simulink model "Advanced_PID"  (R2023a)
settings: Solver=VariableStepAuto  StartTime=0.0  StopTime=100  RelTol=1e-3
model workspace (MAT data in the model file):
  A = [400000 0]
  Ti = 0
libraries: cstblocks x8, slpidlib x4
settings Model: PacingRate=5  Creator=munam  LastModifiedBy=Yuganshu Wadhwa

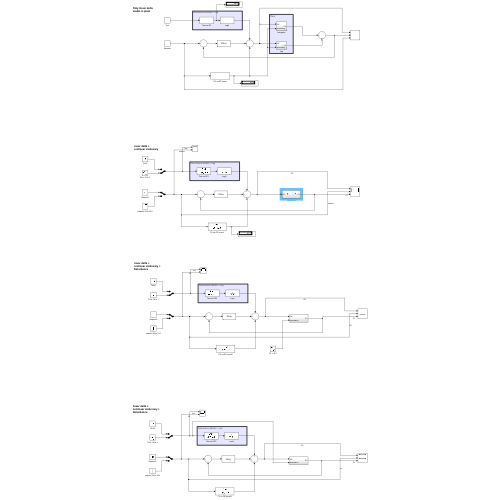
[thumbnail: Simulink's stored preview of the top-level diagram]
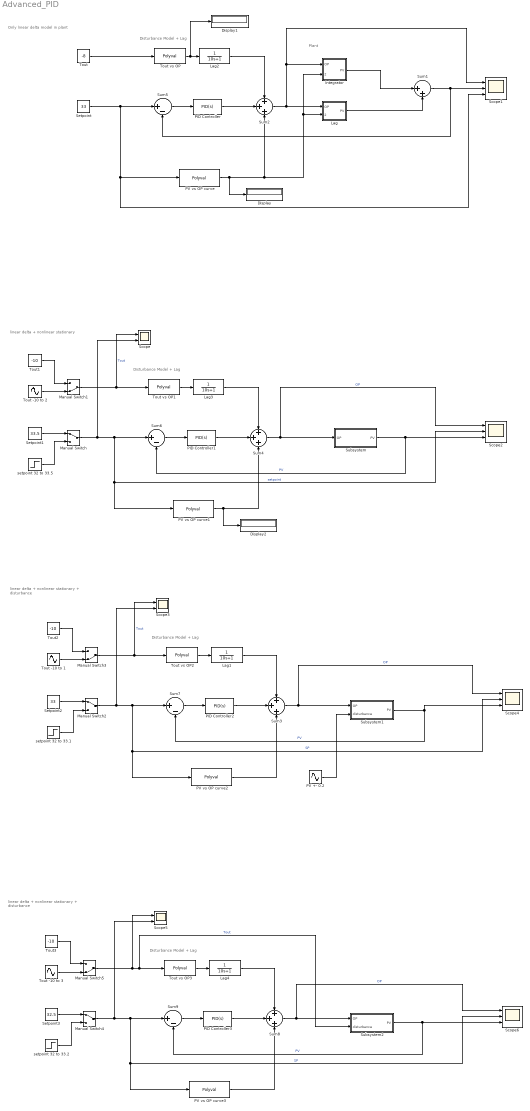
== system Advanced_PID ==
  note: Only linear delta model in plant
  note: Plant
  note: Disturbance Model + Lag
  note: Disturbance Model + Lag
  note: linear delta + nonlinear stationary
  note: linear delta + nonlinear stationary + disturbance
  note: Disturbance Model + Lag
  note: linear delta + nonlinear stationary + disturbance
  note: Disturbance Model + Lag
  Display : Display
  Display1 : Display
  Display2 : Display
  Integrator : Subsystem
  Lag : Subsystem
  Lag{1..4} (4 alike) : TransferFcn  Denominator=[10 1]
  Manual Switch : ManualSwitch
  Manual Switch1 : ManualSwitch  CurrentSetting=0
  Manual Switch2 : ManualSwitch
  Manual Switch3 : ManualSwitch  CurrentSetting=0
  Manual Switch4 : ManualSwitch
  Manual Switch5 : ManualSwitch  CurrentSetting=0
  PID Controller : slpidlib/PID Controller  Controller=PID  Form=Parallel  TimeDomain=Continuous-time  UseExternalTs=off  SampleTime=-1  IntegratorMethod=Forward Euler  FilterMethod=Forward Euler  ControllerParametersSource=internal  P=5  I=2  UseKiTs=off  D=0  N=1  UseFilter=on  TunerSelectOption=Transfer Function Based (PID Tuner App)  InitialConditionSource=internal  InitialConditionForIntegrator=0  InitialConditionForFilter=0  DifferentiatorICPrevScaledInput=0  ExternalReset=none  TrackingMode=off  Kt=1  LimitOutput=off  SatLimitsSource=internal  UpperSaturationLimit=100  LowerSaturationLimit=0  LinearizeAsGain=off  AntiWindupMode=none  Kb=1  LimitIntegrator=off  UpperIntegratorSaturationLimit=inf  LowerIntegratorSaturationLimit=-inf  POutMin=[]  POutMax=[]  IOutMin=[]  IOutMax=[]  DOutMin=[]  DOutMax=[]  NOutMin=[]  NOutMax=[]  SumOutMin=[]  SumOutMax=[]  SaturationOutMin=[]  SaturationOutMax=[]  PParamMin=[]  PParamMax=[]  IParamMin=[]  IParamMax=[]  DParamMin=[]  DParamMax=[]  NParamMin=[]  NParamMax=[]  KbParamMin=[]  KbParamMax=[]  KtParamMin=[]  KtParamMax=[]  KbOutMin=[]  KbOutMax=[]  KtOutMin=[]  KtOutMax=[]  IntegratorOutMin=[]  IntegratorOutMax=[]  FilterOutMin=[]  FilterOutMax=[]  SumI1OutMin=[]  SumI1OutMax=[]  SumI2OutMin=[]  SumI2OutMax=[]  SumI3OutMin=[]  SumI3OutMax=[]  SumI4OutMin=[]  SumI4OutMax=[]  SumDOutMin=[]  SumDOutMax=[]  DifferentiatorOutMin=[]  DifferentiatorOutMax=[]  FilterDiffOutCoefMin=[]  FilterDiffOutCoefMax=[]  ReciprocalOutMin=[]  ReciprocalOutMax=[]  SumDenOutMin=[]  SumDenOutMax=[]  SumNumOutMin=[]  SumNumOutMax=[]  DivideOutMin=[]  DivideOutMax=[]  UdiffTsProdOutMin=[]  UdiffTsProdOutMax=[]  NTsProdOutMin=[]  NTsProdOutMax=[]  UintegralTsProdOutMin=[]  UintegralTsProdOutMax=[]  UngainTsProdOutMin=[]  UngainTsProdOutMax=[]  ClampingZeroOutDataTypeStr=Inherit: Inherit via back propagation  ClampingZeroOutMin=[]  ClampingZeroOutMax=[]  FilterDenConstantOutDataTypeStr=Inherit: Inherit via back propagation  FilterDenConstantOutMin=[]  FilterDenConstantOutMax=[]  PCopyOutDataTypeStr=Inherit: Inherit via back propagation  PCopyOutMin=[]  PCopyOutMax=[]  NCopyOutDataTypeStr=Inherit: Inherit via back propagation  NCopyOutMin=[]  NCopyOutMax=[]  IntegratorContinuousStateAttributes=''  IntegratorStateMustResolveToSignalObject=off  IntegratorRTWStateStorageClass=Auto  FilterContinuousStateAttributes=''  FilterStateMustResolveToSignalObject=off  FilterRTWStateStorageClass=Auto  ParallelPVariant=InternalParameters  IdealPVariant=Disabled  IVariant=InternalParameters  DVariant=InternalParameters  IntegratorVariant=Continuous  SatVariant=Disabled  AWVariant=Passthrough  PCopyVariant=Disabled  TRVariant=Disabled  FdbkBlocksVariant=Forward  IdealPFdbkVariant=Disabled  SatFdbkVariant=Disabled  DerivativeFilterVariant=ContFilter  NVariant=InternalParameters  NCopyVariant=Disabled  FilterICVariant=InternalICsFilter  IntegratorICVariant=InternalICs  ExternalResetVariant=Disabled  TRSumVariant=Passthrough  SumFdbkVariant=Disabled  SumVariant=Sum_PID  TsampFilterVariant=InternalTs  TsampNgainVariant=Passthrough  TsampIntegralVariant=Disabled_SignalSpec  ExternalSaturationOutDataTypeStr=Inherit: Same as second input
  PID Controller1 : slpidlib/PID Controller  Controller=PID  Form=Parallel  TimeDomain=Continuous-time  UseExternalTs=off  SampleTime=-1  IntegratorMethod=Forward Euler  FilterMethod=Forward Euler  ControllerParametersSource=internal  P=5  I=3  UseKiTs=off  D=0  N=1  UseFilter=on  TunerSelectOption=Transfer Function Based (PID Tuner App)  InitialConditionSource=internal  InitialConditionForIntegrator=0  InitialConditionForFilter=0  DifferentiatorICPrevScaledInput=0  ExternalReset=none  TrackingMode=off  Kt=1  LimitOutput=off  SatLimitsSource=internal  UpperSaturationLimit=100  LowerSaturationLimit=0  LinearizeAsGain=off  AntiWindupMode=back-calculation  Kb=1  LimitIntegrator=off  UpperIntegratorSaturationLimit=inf  LowerIntegratorSaturationLimit=-inf  POutMin=[]  POutMax=[]  IOutMin=[]  IOutMax=[]  DOutMin=[]  DOutMax=[]  NOutMin=[]  NOutMax=[]  SumOutMin=[]  SumOutMax=[]  SaturationOutMin=[]  SaturationOutMax=[]  PParamMin=[]  PParamMax=[]  IParamMin=[]  IParamMax=[]  DParamMin=[]  DParamMax=[]  NParamMin=[]  NParamMax=[]  KbParamMin=[]  KbParamMax=[]  KtParamMin=[]  KtParamMax=[]  KbOutMin=[]  KbOutMax=[]  KtOutMin=[]  KtOutMax=[]  IntegratorOutMin=[]  IntegratorOutMax=[]  FilterOutMin=[]  FilterOutMax=[]  SumI1OutMin=[]  SumI1OutMax=[]  SumI2OutMin=[]  SumI2OutMax=[]  SumI3OutMin=[]  SumI3OutMax=[]  SumI4OutMin=[]  SumI4OutMax=[]  SumDOutMin=[]  SumDOutMax=[]  DifferentiatorOutMin=[]  DifferentiatorOutMax=[]  FilterDiffOutCoefMin=[]  FilterDiffOutCoefMax=[]  ReciprocalOutMin=[]  ReciprocalOutMax=[]  SumDenOutMin=[]  SumDenOutMax=[]  SumNumOutMin=[]  SumNumOutMax=[]  DivideOutMin=[]  DivideOutMax=[]  UdiffTsProdOutMin=[]  UdiffTsProdOutMax=[]  NTsProdOutMin=[]  NTsProdOutMax=[]  UintegralTsProdOutMin=[]  UintegralTsProdOutMax=[]  UngainTsProdOutMin=[]  UngainTsProdOutMax=[]  ClampingZeroOutDataTypeStr=Inherit: Inherit via back propagation  ClampingZeroOutMin=[]  ClampingZeroOutMax=[]  FilterDenConstantOutDataTypeStr=Inherit: Inherit via back propagation  FilterDenConstantOutMin=[]  FilterDenConstantOutMax=[]  PCopyOutDataTypeStr=Inherit: Inherit via back propagation  PCopyOutMin=[]  PCopyOutMax=[]  NCopyOutDataTypeStr=Inherit: Inherit via back propagation  NCopyOutMin=[]  NCopyOutMax=[]  IntegratorContinuousStateAttributes=''  IntegratorStateMustResolveToSignalObject=off  IntegratorRTWStateStorageClass=Auto  FilterContinuousStateAttributes=''  FilterStateMustResolveToSignalObject=off  FilterRTWStateStorageClass=Auto  ParallelPVariant=InternalParameters  IdealPVariant=Disabled  IVariant=InternalParameters  DVariant=InternalParameters  IntegratorVariant=Continuous  SatVariant=Disabled  AWVariant=Passthrough  PCopyVariant=Disabled  TRVariant=Disabled  FdbkBlocksVariant=Forward  IdealPFdbkVariant=Disabled  SatFdbkVariant=Disabled  DerivativeFilterVariant=ContFilter  NVariant=InternalParameters  NCopyVariant=Disabled  FilterICVariant=InternalICsFilter  IntegratorICVariant=InternalICs  ExternalResetVariant=Disabled  TRSumVariant=Passthrough  SumFdbkVariant=Disabled  SumVariant=Sum_PID  TsampFilterVariant=InternalTs  TsampNgainVariant=Passthrough  TsampIntegralVariant=Disabled_SignalSpec  ExternalSaturationOutDataTypeStr=Inherit: Same as second input
  PID Controller2 : slpidlib/PID Controller  Controller=PID  Form=Parallel  TimeDomain=Continuous-time  UseExternalTs=off  SampleTime=-1  IntegratorMethod=Forward Euler  FilterMethod=Forward Euler  ControllerParametersSource=internal  P=5  I=3  UseKiTs=off  D=0  N=1  UseFilter=on  TunerSelectOption=Transfer Function Based (PID Tuner App)  InitialConditionSource=internal  InitialConditionForIntegrator=0  InitialConditionForFilter=0  DifferentiatorICPrevScaledInput=0  ExternalReset=none  TrackingMode=off  Kt=1  LimitOutput=off  SatLimitsSource=internal  UpperSaturationLimit=100  LowerSaturationLimit=0  LinearizeAsGain=off  AntiWindupMode=back-calculation  Kb=1  LimitIntegrator=off  UpperIntegratorSaturationLimit=inf  LowerIntegratorSaturationLimit=-inf  POutMin=[]  POutMax=[]  IOutMin=[]  IOutMax=[]  DOutMin=[]  DOutMax=[]  NOutMin=[]  NOutMax=[]  SumOutMin=[]  SumOutMax=[]  SaturationOutMin=[]  SaturationOutMax=[]  PParamMin=[]  PParamMax=[]  IParamMin=[]  IParamMax=[]  DParamMin=[]  DParamMax=[]  NParamMin=[]  NParamMax=[]  KbParamMin=[]  KbParamMax=[]  KtParamMin=[]  KtParamMax=[]  KbOutMin=[]  KbOutMax=[]  KtOutMin=[]  KtOutMax=[]  IntegratorOutMin=[]  IntegratorOutMax=[]  FilterOutMin=[]  FilterOutMax=[]  SumI1OutMin=[]  SumI1OutMax=[]  SumI2OutMin=[]  SumI2OutMax=[]  SumI3OutMin=[]  SumI3OutMax=[]  SumI4OutMin=[]  SumI4OutMax=[]  SumDOutMin=[]  SumDOutMax=[]  DifferentiatorOutMin=[]  DifferentiatorOutMax=[]  FilterDiffOutCoefMin=[]  FilterDiffOutCoefMax=[]  ReciprocalOutMin=[]  ReciprocalOutMax=[]  SumDenOutMin=[]  SumDenOutMax=[]  SumNumOutMin=[]  SumNumOutMax=[]  DivideOutMin=[]  DivideOutMax=[]  UdiffTsProdOutMin=[]  UdiffTsProdOutMax=[]  NTsProdOutMin=[]  NTsProdOutMax=[]  UintegralTsProdOutMin=[]  UintegralTsProdOutMax=[]  UngainTsProdOutMin=[]  UngainTsProdOutMax=[]  ClampingZeroOutDataTypeStr=Inherit: Inherit via back propagation  ClampingZeroOutMin=[]  ClampingZeroOutMax=[]  FilterDenConstantOutDataTypeStr=Inherit: Inherit via back propagation  FilterDenConstantOutMin=[]  FilterDenConstantOutMax=[]  PCopyOutDataTypeStr=Inherit: Inherit via back propagation  PCopyOutMin=[]  PCopyOutMax=[]  NCopyOutDataTypeStr=Inherit: Inherit via back propagation  NCopyOutMin=[]  NCopyOutMax=[]  IntegratorContinuousStateAttributes=''  IntegratorStateMustResolveToSignalObject=off  IntegratorRTWStateStorageClass=Auto  FilterContinuousStateAttributes=''  FilterStateMustResolveToSignalObject=off  FilterRTWStateStorageClass=Auto  ParallelPVariant=InternalParameters  IdealPVariant=Disabled  IVariant=InternalParameters  DVariant=InternalParameters  IntegratorVariant=Continuous  SatVariant=Disabled  AWVariant=Passthrough  PCopyVariant=Disabled  TRVariant=Disabled  FdbkBlocksVariant=Forward  IdealPFdbkVariant=Disabled  SatFdbkVariant=Disabled  DerivativeFilterVariant=ContFilter  NVariant=InternalParameters  NCopyVariant=Disabled  FilterICVariant=InternalICsFilter  IntegratorICVariant=InternalICs  ExternalResetVariant=Disabled  TRSumVariant=Passthrough  SumFdbkVariant=Disabled  SumVariant=Sum_PID  TsampFilterVariant=InternalTs  TsampNgainVariant=Passthrough  TsampIntegralVariant=Disabled_SignalSpec  ExternalSaturationOutDataTypeStr=Inherit: Same as second input
  PID Controller3 : slpidlib/PID Controller  Controller=PID  Form=Parallel  TimeDomain=Continuous-time  UseExternalTs=off  SampleTime=-1  IntegratorMethod=Forward Euler  FilterMethod=Forward Euler  ControllerParametersSource=internal  P=5  I=3  UseKiTs=off  D=0  N=1  UseFilter=on  TunerSelectOption=Transfer Function Based (PID Tuner App)  InitialConditionSource=internal  InitialConditionForIntegrator=0  InitialConditionForFilter=0  DifferentiatorICPrevScaledInput=0  ExternalReset=none  TrackingMode=off  Kt=1  LimitOutput=off  SatLimitsSource=internal  UpperSaturationLimit=100  LowerSaturationLimit=0  LinearizeAsGain=off  AntiWindupMode=back-calculation  Kb=1  LimitIntegrator=off  UpperIntegratorSaturationLimit=inf  LowerIntegratorSaturationLimit=-inf  POutMin=[]  POutMax=[]  IOutMin=[]  IOutMax=[]  DOutMin=[]  DOutMax=[]  NOutMin=[]  NOutMax=[]  SumOutMin=[]  SumOutMax=[]  SaturationOutMin=[]  SaturationOutMax=[]  PParamMin=[]  PParamMax=[]  IParamMin=[]  IParamMax=[]  DParamMin=[]  DParamMax=[]  NParamMin=[]  NParamMax=[]  KbParamMin=[]  KbParamMax=[]  KtParamMin=[]  KtParamMax=[]  KbOutMin=[]  KbOutMax=[]  KtOutMin=[]  KtOutMax=[]  IntegratorOutMin=[]  IntegratorOutMax=[]  FilterOutMin=[]  FilterOutMax=[]  SumI1OutMin=[]  SumI1OutMax=[]  SumI2OutMin=[]  SumI2OutMax=[]  SumI3OutMin=[]  SumI3OutMax=[]  SumI4OutMin=[]  SumI4OutMax=[]  SumDOutMin=[]  SumDOutMax=[]  DifferentiatorOutMin=[]  DifferentiatorOutMax=[]  FilterDiffOutCoefMin=[]  FilterDiffOutCoefMax=[]  ReciprocalOutMin=[]  ReciprocalOutMax=[]  SumDenOutMin=[]  SumDenOutMax=[]  SumNumOutMin=[]  SumNumOutMax=[]  DivideOutMin=[]  DivideOutMax=[]  UdiffTsProdOutMin=[]  UdiffTsProdOutMax=[]  NTsProdOutMin=[]  NTsProdOutMax=[]  UintegralTsProdOutMin=[]  UintegralTsProdOutMax=[]  UngainTsProdOutMin=[]  UngainTsProdOutMax=[]  ClampingZeroOutDataTypeStr=Inherit: Inherit via back propagation  ClampingZeroOutMin=[]  ClampingZeroOutMax=[]  FilterDenConstantOutDataTypeStr=Inherit: Inherit via back propagation  FilterDenConstantOutMin=[]  FilterDenConstantOutMax=[]  PCopyOutDataTypeStr=Inherit: Inherit via back propagation  PCopyOutMin=[]  PCopyOutMax=[]  NCopyOutDataTypeStr=Inherit: Inherit via back propagation  NCopyOutMin=[]  NCopyOutMax=[]  IntegratorContinuousStateAttributes=''  IntegratorStateMustResolveToSignalObject=off  IntegratorRTWStateStorageClass=Auto  FilterContinuousStateAttributes=''  FilterStateMustResolveToSignalObject=off  FilterRTWStateStorageClass=Auto  ParallelPVariant=InternalParameters  IdealPVariant=Disabled  IVariant=InternalParameters  DVariant=InternalParameters  IntegratorVariant=Continuous  SatVariant=Disabled  AWVariant=Passthrough  PCopyVariant=Disabled  TRVariant=Disabled  FdbkBlocksVariant=Forward  IdealPFdbkVariant=Disabled  SatFdbkVariant=Disabled  DerivativeFilterVariant=ContFilter  NVariant=InternalParameters  NCopyVariant=Disabled  FilterICVariant=InternalICsFilter  IntegratorICVariant=InternalICs  ExternalResetVariant=Disabled  TRSumVariant=Passthrough  SumFdbkVariant=Disabled  SumVariant=Sum_PID  TsampFilterVariant=InternalTs  TsampNgainVariant=Passthrough  TsampIntegralVariant=Disabled_SignalSpec  ExternalSaturationOutDataTypeStr=Inherit: Same as second input
  PV +- 0.2 : Sin  Amplitude=0.2  Frequency=(3.472e-05)*2*pi  SampleTime=0
  PV vs OP curve{,1..3} (4 alike) : Polyval  Coefs=[ +20.075, -1284.7, 20570]
  Scope : Scope  NumInputPorts=2
  Scope{1..2,4,6} (4 alike) : Scope  NumInputPorts=3
  Scope3 : Scope  NumInputPorts=2
  Scope5 : Scope  NumInputPorts=2
  Setpoint : Constant  Value=33
  Setpoint1 : Constant  Value=33.5
  Setpoint2 : Constant  Value=33
  Setpoint3 : Constant  Value=32.5
  Subsystem : Subsystem
  Subsystem1 : Subsystem
  Subsystem2 : Subsystem
  Sum1 : Sum  Inputs=|++
  Sum{2..4,8} (4 alike) : Sum  Inputs=+++
  Sum{5..7,9} (4 alike) : Sum  Inputs=|+-
  Tout : Constant  Value=-8
  Tout -10 to 1 : Sin  Amplitude=6  Bias=-4  Frequency=(3.472e-05)*2*pi  SampleTime=0
  Tout -10 to 2 : Sin  Amplitude=6  Bias=-4  Frequency=(3.472e-05)*2*pi  SampleTime=0
  Tout -10 to 3 : Sin  Amplitude=6  Bias=-4  Frequency=(3.472e-05)*2*pi  SampleTime=0
  Tout vs OP{,1..3} (4 alike) : Polyval  Coefs=[ +0.5285, +0.2364, +16.302 ]
  Tout1 : Constant  Value=-10
  Tout2 : Constant  Value=-10
  Tout3 : Constant  Value=-10
  setpoint 32 to 33.1 : Step  Time=100  Before=32  After=33.5  SampleTime=0
  setpoint 32 to 33.2 : Step  Time=100  Before=32  After=33.5  SampleTime=0
  setpoint 32 to 33.5 : Step  Time=100  Before=32  After=33.5  SampleTime=0
  wires:
  Integrator/1(PV) -> Sum1/1
  Tout vs OP/1 -> Display1/1, Lag2/1
  Sum1/1 -> Scope1/2, Sum5/2
  Lag/1(PV) -> Sum1/2
  Tout/1 -> Tout vs OP/1
  Sum2/1 -> Scope1/1, Integrator/1(OP), Lag/1(OP)
  Setpoint/1 -> Sum5/1, PV vs OP curve/1, Scope1/3
  Sum5/1 -> PID Controller/1
  PV vs OP curve/1 -> Display/1, Sum2/3, Integrator/2(scheduling), Lag/2(scheduling)
  PID Controller/1 -> Sum2/2
  Lag2/1 -> Sum2/1
  PV vs OP curve1/1 -> Display2/1, Sum4/3
  Manual Switch/1 -> Scope/2, PV vs OP curve1/1, Scope2/2, Sum6/1  "setpoint"
  Subsystem/1(PV) -> Scope2/3, Sum6/2  "PV"
  PID Controller1/1 -> Sum4/2
  Manual Switch1/1 -> Scope/1, Tout vs OP1/1  "Tout"
  Sum6/1 -> PID Controller1/1
  Tout vs OP1/1 -> Lag3/1
  Sum4/1 -> Scope2/1, Subsystem/1(OP)  "OP"
  Lag3/1 -> Sum4/1
  Setpoint1/1 -> Manual Switch/1
  setpoint 32 to 33.5/1 -> Manual Switch/2
  Tout -10 to 2/1 -> Manual Switch1/2
  Tout1/1 -> Manual Switch1/1
  Manual Switch3/1 -> Scope3/1, Tout vs OP2/1  "Tout"
  setpoint 32 to 33.1/1 -> Manual Switch2/2
  Sum3/1 -> Scope4/1, Subsystem1/1(OP)  "OP"
  PID Controller2/1 -> Sum3/2
  Subsystem1/1(PV) -> Scope4/3, Sum7/2  "PV"
  Sum7/1 -> PID Controller2/1
  Manual Switch2/1 -> Scope3/2, PV vs OP curve2/1, Scope4/2, Sum7/1  "SP"
  Setpoint2/1 -> Manual Switch2/1
  Tout -10 to 1/1 -> Manual Switch3/2
  PV vs OP curve2/1 -> Sum3/3
  Tout vs OP2/1 -> Lag1/1
  Tout2/1 -> Manual Switch3/1
  Lag1/1 -> Sum3/1
  Lag4/1 -> Sum8/1
  Tout vs OP3/1 -> Lag4/1
  Tout -10 to 3/1 -> Manual Switch5/2
  Tout3/1 -> Manual Switch5/1
  Sum9/1 -> PID Controller3/1
  PV vs OP curve3/1 -> Sum8/3
  Setpoint3/1 -> Manual Switch4/1
  Sum8/1 -> Scope6/1, Subsystem2/1(OP)  "OP"
  Manual Switch4/1 -> Scope5/2, PV vs OP curve3/1, Scope6/2, Sum9/1  "SP"
  Subsystem2/1(PV) -> Scope6/3, Sum9/2  "PV"
  setpoint 32 to 33.2/1 -> Manual Switch4/2
  Manual Switch5/1 -> Scope5/1, Subsystem2/2(disturbance), Tout vs OP3/1  "Tout"
  PID Controller3/1 -> Sum8/2
  PV +- 0.2/1 -> Subsystem1/2(disturbance)

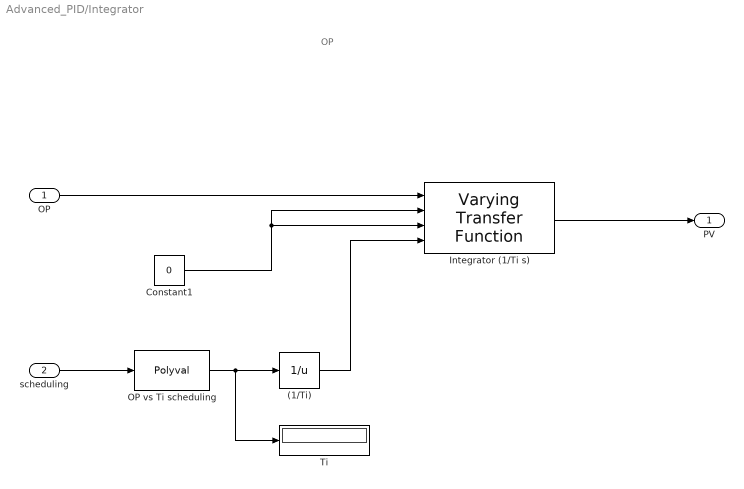
== system Advanced_PID/Integrator ==
  note: OP
  OP : Inport
  scheduling : Inport  Port=2
  (1/Ti) : Math  Operator=reciprocal
  Constant1 : Constant  Value=0
  Integrator (1/Ti s) : cstblocks/Linear Parameter Varying/Varying Transfer Function  N=1  Feedthrough=on
  OP vs Ti scheduling : Polyval  Coefs=[ +511.04, -14301, +405369 ]
  Ti : Display
  PV : Outport
  wires:
  OP/1 -> Integrator (1/Ti s)/1
  Constant1/1 -> Integrator (1/Ti s)/3, Integrator (1/Ti s)/2
  OP vs Ti scheduling/1 -> Ti/1, (1/Ti)/1
  Integrator (1/Ti s)/1 -> PV/1
  (1/Ti)/1 -> Integrator (1/Ti s)/4
  scheduling/1 -> OP vs Ti scheduling/1

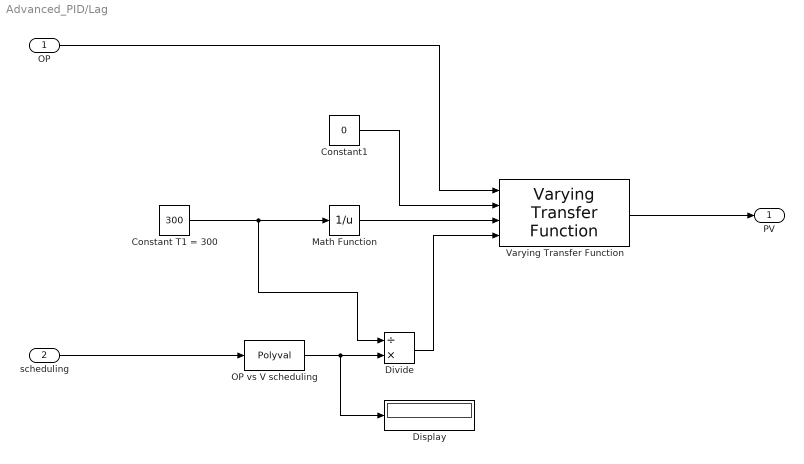
== system Advanced_PID/Lag ==
  OP : Inport
  scheduling : Inport  Port=2
  Constant T1 = 300 : Constant  Value=300
  Constant1 : Constant  Value=0
  Display : Display
  Divide : Product  Inputs=/*
  Math Function : Math  Operator=reciprocal
  OP vs V scheduling : Polyval  Coefs="[  -3e-7, +8e-5, -0.0065, 0.1944 ]"
  Varying Transfer Function : cstblocks/Linear Parameter Varying/Varying Transfer Function  N=1  Feedthrough=on
  PV : Outport
  wires:
  Divide/1 -> Varying Transfer Function/4
  Constant T1 = 300/1 -> Math Function/1, Divide/1
  Constant1/1 -> Varying Transfer Function/2
  OP/1 -> Varying Transfer Function/1
  OP vs V scheduling/1 -> Display/1, Divide/2
  Math Function/1 -> Varying Transfer Function/3
  Varying Transfer Function/1 -> PV/1
  scheduling/1 -> OP vs V scheduling/1

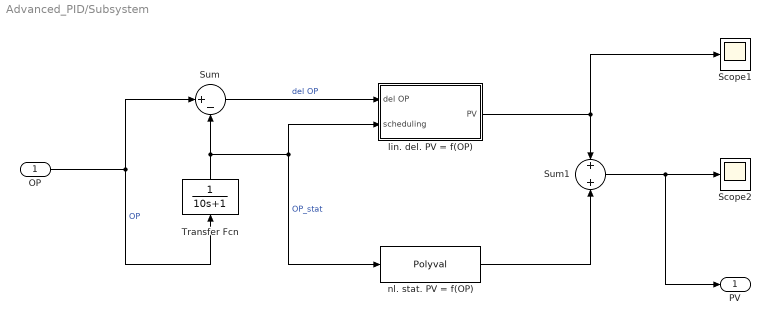
== system Advanced_PID/Subsystem ==
  OP : Inport
  Scope1 : Scope
  Scope2 : Scope
  Sum : Sum  Inputs=|+-
  Sum1 : Sum  Inputs=+|+
  Transfer Fcn : TransferFcn  Denominator=[10 1]
  "lin. del. PV = f(OP) " : Subsystem
  nl. stat. PV = f(OP) : Polyval  Coefs=[ -0.0004, +0.0693, +30.896 ]
  PV : Outport
  wires:
  nl. stat. PV = f(OP)/1 -> Sum1/2
  "lin. del. PV = f(OP) "/1(PV) -> Scope1/1, Sum1/1
  Sum1/1 -> Scope2/1, PV/1
  Sum/1 -> "lin. del. PV = f(OP) "/1(del OP)  "del OP"
  OP/1 -> Sum/1, Transfer Fcn/1  "OP"
  Transfer Fcn/1 -> nl. stat. PV = f(OP)/1, "lin. del. PV = f(OP) "/2(scheduling), Sum/2  "OP_stat"

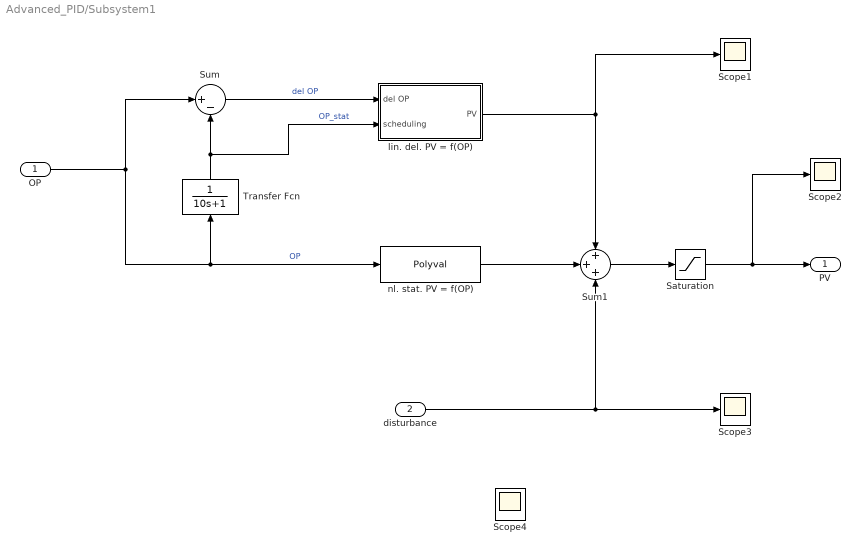
== system Advanced_PID/Subsystem1 ==
  OP : Inport
  disturbance : Inport  Port=2
  Saturation : Saturate  UpperLimit=33.9  LowerLimit=31.7
  Scope{1..4} (4 alike) : Scope
  Sum : Sum  Inputs=|+-
  Sum1 : Sum  Inputs=+++
  Transfer Fcn : TransferFcn  Denominator=[10 1]
  "lin. del. PV = f(OP) " : Subsystem
  nl. stat. PV = f(OP) : Polyval  Coefs=[ -0.0004, +0.0693, +30.896 ]
  PV : Outport
  wires:
  nl. stat. PV = f(OP)/1 -> Sum1/2
  "lin. del. PV = f(OP) "/1(PV) -> Scope1/1, Sum1/1
  Saturation/1 -> Scope2/1, PV/1
  Sum/1 -> "lin. del. PV = f(OP) "/1(del OP)  "del OP"
  OP/1 -> Sum/1, Transfer Fcn/1, nl. stat. PV = f(OP)/1  "OP"
  Transfer Fcn/1 -> "lin. del. PV = f(OP) "/2(scheduling), Sum/2  "OP_stat"
  Sum1/1 -> Saturation/1
  disturbance/1 -> Sum1/3, Scope3/1

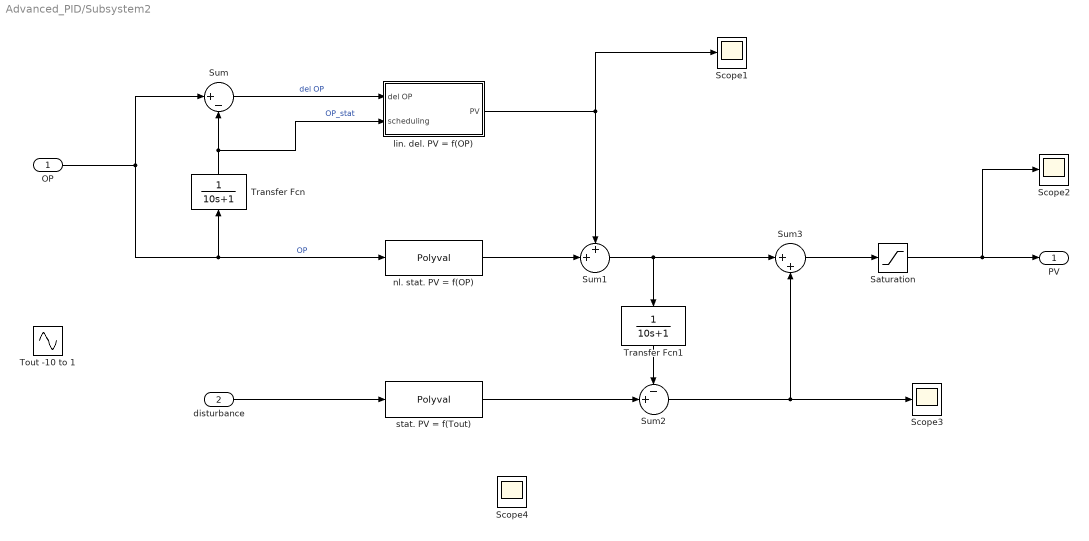
== system Advanced_PID/Subsystem2 ==
  OP : Inport
  disturbance : Inport  Port=2
  Saturation : Saturate  UpperLimit=33.9  LowerLimit=31.7
  Scope{1..4} (4 alike) : Scope
  Sum : Sum  Inputs=|+-
  Sum1 : Sum  Inputs=++|
  Sum2 : Sum  Inputs=-+|
  Sum3 : Sum  Inputs=|++
  Tout -10 to 1 : Sin  Amplitude=0.2  Frequency=(3.472e-05)*2*pi  SampleTime=0
  Transfer Fcn : TransferFcn  Denominator=[10 1]
  Transfer Fcn1 : TransferFcn  Denominator=[10 1]
  "lin. del. PV = f(OP) " : Subsystem
  nl. stat. PV = f(OP) : Polyval  Coefs=[ -0.0004, +0.0693, +30.896 ]
  stat. PV = f(Tout) : Polyval  Coefs=[ -0.1576, +31.9999]
  PV : Outport
  wires:
  nl. stat. PV = f(OP)/1 -> Sum1/2
  "lin. del. PV = f(OP) "/1(PV) -> Scope1/1, Sum1/1
  Saturation/1 -> Scope2/1, PV/1
  Sum/1 -> "lin. del. PV = f(OP) "/1(del OP)  "del OP"
  OP/1 -> Sum/1, Transfer Fcn/1, nl. stat. PV = f(OP)/1  "OP"
  Transfer Fcn/1 -> "lin. del. PV = f(OP) "/2(scheduling), Sum/2  "OP_stat"
  disturbance/1 -> stat. PV = f(Tout)/1
  stat. PV = f(Tout)/1 -> Sum2/2
  Sum2/1 -> Sum3/2, Scope3/1
  Sum1/1 -> Transfer Fcn1/1, Sum3/1
  Transfer Fcn1/1 -> Sum2/1
  Sum3/1 -> Saturation/1

== system Advanced_PID/Subsystem/lin. del. PV = f(OP)  ==
  del OP : Inport
  scheduling : Inport  Port=2
  Integrator : Subsystem
  Lag : Subsystem
  Sum : Sum  Inputs=+|+
  PV : Outport
  wires:
  Lag/1(PV) -> Sum/2
  Sum/1 -> PV/1
  scheduling/1 -> Integrator/2(scheduling), Lag/2(scheduling)
  del OP/1 -> Lag/1(OP), Integrator/1(OP)
  Integrator/1(PV) -> Sum/1

== system Advanced_PID/Subsystem1/lin. del. PV = f(OP)  ==
  del OP : Inport
  scheduling : Inport  Port=2
  Integrator : Subsystem
  Lag : Subsystem
  Sum : Sum  Inputs=+|+
  PV : Outport
  wires:
  Lag/1(PV) -> Sum/2
  Sum/1 -> PV/1
  scheduling/1 -> Integrator/2(scheduling), Lag/2(scheduling)
  del OP/1 -> Lag/1(OP), Integrator/1(OP)
  Integrator/1(PV) -> Sum/1

== system Advanced_PID/Subsystem2/lin. del. PV = f(OP)  ==
  del OP : Inport
  scheduling : Inport  Port=2
  Integrator : Subsystem
  Lag : Subsystem
  Sum : Sum  Inputs=+|+
  PV : Outport
  wires:
  Lag/1(PV) -> Sum/2
  Sum/1 -> PV/1
  scheduling/1 -> Integrator/2(scheduling), Lag/2(scheduling)
  del OP/1 -> Lag/1(OP), Integrator/1(OP)
  Integrator/1(PV) -> Sum/1

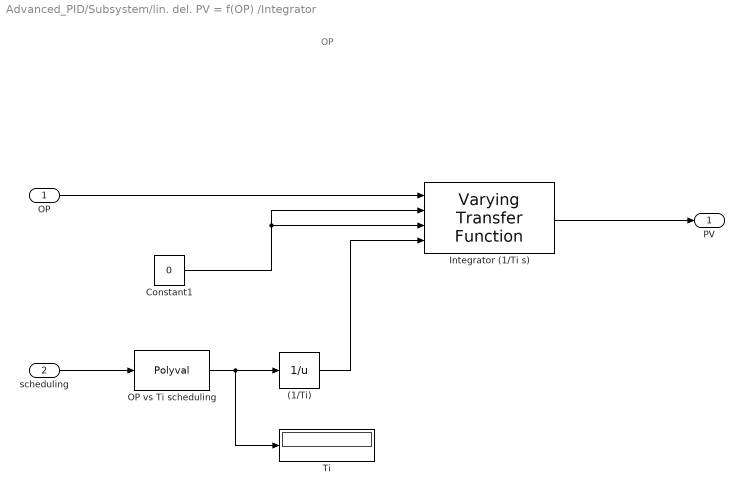
== system Advanced_PID/Subsystem/lin. del. PV = f(OP) /Integrator ==
  note: OP
  OP : Inport
  scheduling : Inport  Port=2
  (1/Ti) : Math  Operator=reciprocal
  Constant1 : Constant  Value=0
  Integrator (1/Ti s) : cstblocks/Linear Parameter Varying/Varying Transfer Function  N=1  Feedthrough=on
  OP vs Ti scheduling : Polyval  Coefs=[ +0.3812, -72.91, +4942.1, -110789, +1e+06 ]
  Ti : Display
  PV : Outport
  wires:
  OP/1 -> Integrator (1/Ti s)/1
  Constant1/1 -> Integrator (1/Ti s)/3, Integrator (1/Ti s)/2
  OP vs Ti scheduling/1 -> Ti/1, (1/Ti)/1
  Integrator (1/Ti s)/1 -> PV/1
  (1/Ti)/1 -> Integrator (1/Ti s)/4
  scheduling/1 -> OP vs Ti scheduling/1

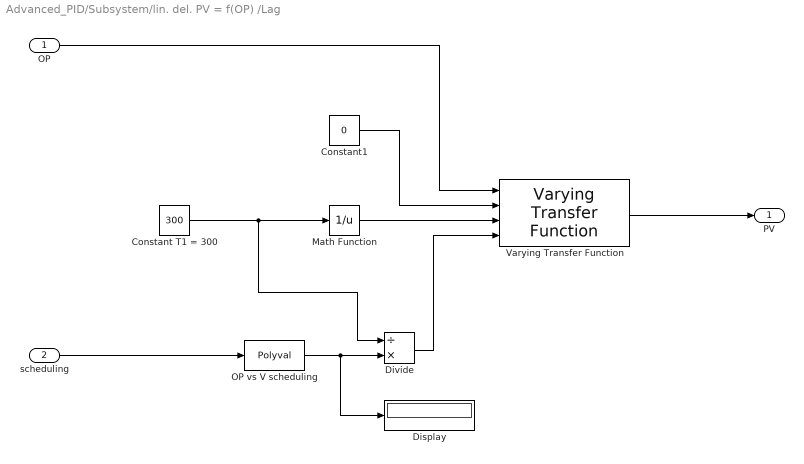
== system Advanced_PID/Subsystem/lin. del. PV = f(OP) /Lag ==
  OP : Inport
  scheduling : Inport  Port=2
  Constant T1 = 300 : Constant  Value=300
  Constant1 : Constant  Value=0
  Display : Display
  Divide : Product  Inputs=/*
  Math Function : Math  Operator=reciprocal
  OP vs V scheduling : Polyval  Coefs="[  -3e-7, +8e-5, -0.0065, 0.1944 ]"
  Varying Transfer Function : cstblocks/Linear Parameter Varying/Varying Transfer Function  N=1  Feedthrough=on
  PV : Outport
  wires:
  Divide/1 -> Varying Transfer Function/4
  Constant T1 = 300/1 -> Math Function/1, Divide/1
  Constant1/1 -> Varying Transfer Function/2
  OP/1 -> Varying Transfer Function/1
  OP vs V scheduling/1 -> Display/1, Divide/2
  Math Function/1 -> Varying Transfer Function/3
  Varying Transfer Function/1 -> PV/1
  scheduling/1 -> OP vs V scheduling/1

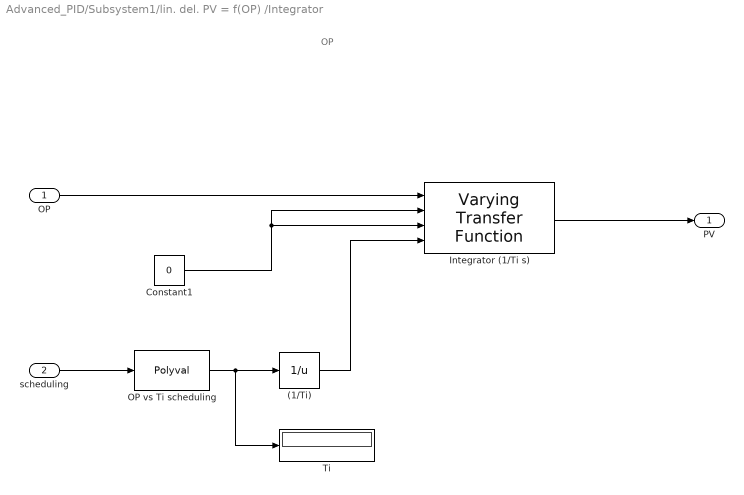
== system Advanced_PID/Subsystem1/lin. del. PV = f(OP) /Integrator ==
  note: OP
  OP : Inport
  scheduling : Inport  Port=2
  (1/Ti) : Math  Operator=reciprocal
  Constant1 : Constant  Value=0
  Integrator (1/Ti s) : cstblocks/Linear Parameter Varying/Varying Transfer Function  N=1  Feedthrough=on
  OP vs Ti scheduling : Polyval  Coefs=[ +0.3812, -72.91, +4942.1, -110789, +1e+06 ]
  Ti : Display
  PV : Outport
  wires:
  OP/1 -> Integrator (1/Ti s)/1
  Constant1/1 -> Integrator (1/Ti s)/3, Integrator (1/Ti s)/2
  OP vs Ti scheduling/1 -> Ti/1, (1/Ti)/1
  Integrator (1/Ti s)/1 -> PV/1
  (1/Ti)/1 -> Integrator (1/Ti s)/4
  scheduling/1 -> OP vs Ti scheduling/1

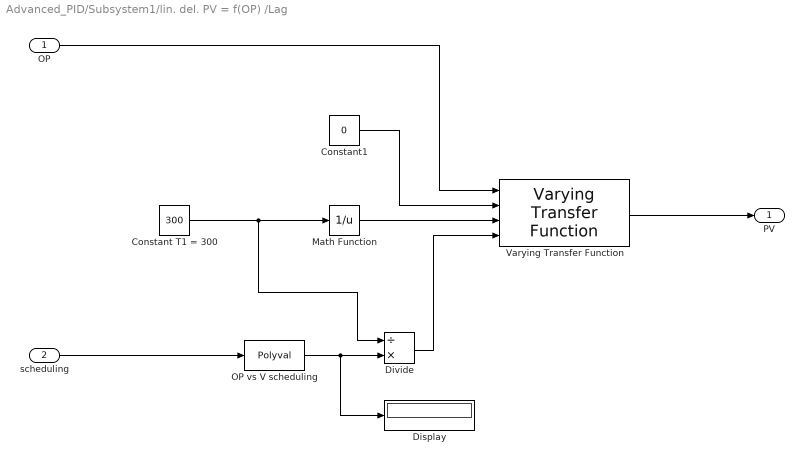
== system Advanced_PID/Subsystem1/lin. del. PV = f(OP) /Lag ==
  OP : Inport
  scheduling : Inport  Port=2
  Constant T1 = 300 : Constant  Value=300
  Constant1 : Constant  Value=0
  Display : Display
  Divide : Product  Inputs=/*
  Math Function : Math  Operator=reciprocal
  OP vs V scheduling : Polyval  Coefs="[  -3e-7, +8e-5, -0.0065, 0.1944 ]"
  Varying Transfer Function : cstblocks/Linear Parameter Varying/Varying Transfer Function  N=1  Feedthrough=on
  PV : Outport
  wires:
  Divide/1 -> Varying Transfer Function/4
  Constant T1 = 300/1 -> Math Function/1, Divide/1
  Constant1/1 -> Varying Transfer Function/2
  OP/1 -> Varying Transfer Function/1
  OP vs V scheduling/1 -> Display/1, Divide/2
  Math Function/1 -> Varying Transfer Function/3
  Varying Transfer Function/1 -> PV/1
  scheduling/1 -> OP vs V scheduling/1

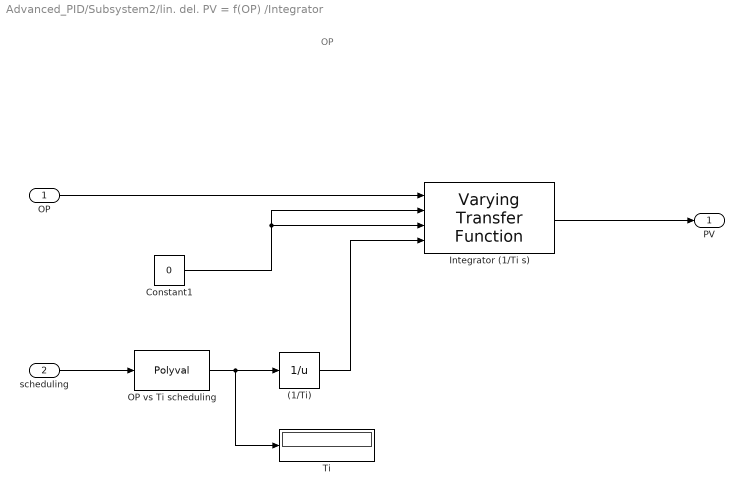
== system Advanced_PID/Subsystem2/lin. del. PV = f(OP) /Integrator ==
  note: OP
  OP : Inport
  scheduling : Inport  Port=2
  (1/Ti) : Math  Operator=reciprocal
  Constant1 : Constant  Value=0
  Integrator (1/Ti s) : cstblocks/Linear Parameter Varying/Varying Transfer Function  N=1  Feedthrough=on
  OP vs Ti scheduling : Polyval  Coefs=[ +0.3812, -72.91, +4942.1, -110789, +1e+06 ]
  Ti : Display
  PV : Outport
  wires:
  OP/1 -> Integrator (1/Ti s)/1
  Constant1/1 -> Integrator (1/Ti s)/3, Integrator (1/Ti s)/2
  OP vs Ti scheduling/1 -> Ti/1, (1/Ti)/1
  Integrator (1/Ti s)/1 -> PV/1
  (1/Ti)/1 -> Integrator (1/Ti s)/4
  scheduling/1 -> OP vs Ti scheduling/1

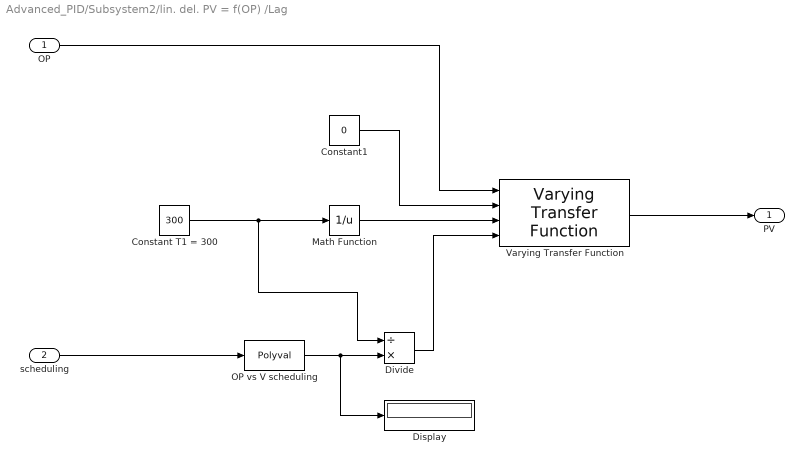
== system Advanced_PID/Subsystem2/lin. del. PV = f(OP) /Lag ==
  OP : Inport
  scheduling : Inport  Port=2
  Constant T1 = 300 : Constant  Value=300
  Constant1 : Constant  Value=0
  Display : Display
  Divide : Product  Inputs=/*
  Math Function : Math  Operator=reciprocal
  OP vs V scheduling : Polyval  Coefs="[  -3e-7, +8e-5, -0.0065, 0.1944 ]"
  Varying Transfer Function : cstblocks/Linear Parameter Varying/Varying Transfer Function  N=1  Feedthrough=on
  PV : Outport
  wires:
  Divide/1 -> Varying Transfer Function/4
  Constant T1 = 300/1 -> Math Function/1, Divide/1
  Constant1/1 -> Varying Transfer Function/2
  OP/1 -> Varying Transfer Function/1
  OP vs V scheduling/1 -> Display/1, Divide/2
  Math Function/1 -> Varying Transfer Function/3
  Varying Transfer Function/1 -> PV/1
  scheduling/1 -> OP vs V scheduling/1
